simulink model "CDPR_simulation"  (R2021b)
settings: Solver=VariableStepAuto  StartTime=0.0  StopTime=40.0  RelTol=1e-3
values from neighbouring files (symbols this model uses):
  a = [-2.0 2.0 ... (first row only)    [init.m]
  A_p = [0  1   0  0   0  0 ... (first row only)    [init.m]
  b = [-0.05  0.05 ... (first row only)    [init.m]
  B_p = [0     0     0 ... (first row only)    [init.m]
  Clarke = 2/3*[1 -1/2       -1/2 ... (first row only)    [motor_init.m]
  epsilon_1 = 1e-17    [init.m]
  epsilon_2 = 1e-17    [init.m]
  f_max = 60*ones(m,1)    [init.m]
  f_min = 2*ones(m,1)    [init.m]
  f_ref = 0.5*(f_min+f_max)    [init.m]
  fourier_coeff_a = [ 0.08333    0.00000     0.00000 ... (first row only)    [motor_init.m]
  fourier_coeff_b = [-1.23020    0.60792     0.60792 ... (first row only)    [motor_init.m]
  J_m_inv = 1000*1/J_m    (= 41564.487302)    [motor_init.m]
  K_e = 0.052    [motor_init.m]
  k_spring = diag(200*ones(m,1))    [init.m]
  k_spring_inv = inv(k_spring)    [init.m]
  l_0 = inverseKinematics(a, b, x, m)    [init.m]
  L_m = 8.97e-6    (= 8.97e-06)    [motor_init.m]
  m = 4    [init.m]
  n_pole_pairs = n_poles/2    (= 7)    [motor_init.m]
  R_m = 19.00e-3    (= 0.019)    [motor_init.m]
  r_winch = 60.0e-3    (= 0.06)    [init.m]
  tau = 1e-6    (= 1e-06)    [init.m]
  theta_r_0 = (l_0-k_spring_inv*f_ref)/r_winch    [init.m]
  x_0 = [x(1); 0; x(2); 0; x(3);0]    [init.m]
  xi = 2    [init.m]
(part 2 of 2)

== matlab function CDPR_simulation/Inverse kinematics2/Inverse kinematics ==
  data: a input; l output; b input; pose input; m input
function l = inverseKinematics(a, b, pose, m)
    x     = pose(1);
    y     = pose(2);
    theta = pose(3);

    l = zeros(4,1);
    for i=1:m
        l(i) = norm(a(:,i)-[x;y]-R_z(theta)*b(:,i),2);
    end
end


function R = R_z(theta)
    R = [cos(theta) -sin(theta);
         sin(theta)  cos(theta)];
end

== matlab function CDPR_simulation/Inverse kinematics/Inverse kinematics ==
  data: a input; l output; b input; pose input; m input
function l = inverseKinematics(a, b, pose, m)
    x     = pose(1);
    y     = pose(2);
    theta = pose(3);

    l = zeros(4,1);
    for i=1:m
        l(i) = norm(a(:,i)-[x;y]-R_z(theta)*b(:,i),2);
    end
end


function R = R_z(theta)
    R = [cos(theta) -sin(theta);
         sin(theta)  cos(theta)];
end

== matlab function CDPR_simulation/Structure matrix/Structure matrix calculation ==
  data: u input; A_T output; pose input; b input; m input
function A_T = calculateStructureMatrix(u, pose, b, m)
    theta = pose(3);
    crossProd = zeros(1, 4);
    for i=1:m
        b_rot = R_z(theta)*b(:,i);
        crossProd(i) = b_rot(1)*u(2,i) - b_rot(2)*u(1,i);
    end
    A_T = [u; crossProd]
end

function R = R_z(theta)
    R = [cos(theta) -sin(theta);
         sin(theta)  cos(theta)];
end

== matlab function CDPR_simulation/Motor 1/FOC BLDC/BLDC motor/Subsystem/MATLAB Function ==
  data: a_f input; f_abc output; b_f input; theta_r input
function f_abc  = normalized_back_EMF(a_f,b_f,theta_r)
sa = 0;
sb = 0;
sc = 0;
ca = 0;
cb = 0;
cc = 0;
n = size(a_f,1);

for i = 1:n
%     ca = ca + a(i,1)*cos((i-1)*theta_r);
    cb = cb + a_f(i,2)*cos((i-1)*theta_r);
    cc = cc + a_f(i,3)*cos((i-1)*theta_r); 
end
for i = 1:2:n
    sa = sa + b_f(i,1)*sin(i*theta_r);
    sb = sb + b_f(i,2)*sin(i*theta_r);
    sc = sc + b_f(i,3)*sin(i*theta_r);
end
f_a = ca+sa;
f_b = cb+sb;
f_c = cc+sc;

f_abc = [f_a;f_b;f_c];

== matlab function CDPR_simulation/Motor 1/FOC BLDC/Inverse Park transformation ==
  data: v_q input; v_d input; v_a output; theta_r input; v_b output; v_c output
function [v_a, v_b, v_c] = inverse_park(v_q, v_d, theta_r)
Park_inv = [cos(theta_r)          -sin(theta_r);
            cos(theta_r - 2*pi/3) -sin(theta_r - 2*pi/3);
            cos(theta_r + 2*pi/3) -sin(theta_r + 2*pi/3)];

v_abc = Park_inv*[v_d;v_q];

v_a = v_abc(1);
v_b = v_abc(2);
v_c = v_abc(3);

== matlab function CDPR_simulation/Motor 1/FOC BLDC/Park transformation ==
  data: i_alphabeta input; i_qd output; theta_r input
function i_qd = park(i_alphabeta, theta_r)
Park = [-sin(theta_r) cos(theta_r);
         cos(theta_r) sin(theta_r)];
i_qd = Park*i_alphabeta;

== matlab function CDPR_simulation/Force distribution/Force distribution calculation ==
  data: A_T input; f input; f_d output; f_min input; f_max input; f_ref input; w input; m input
function f_d = forceQP(A_T, f, f_min, f_max, f_ref, w, m)
    coder.extrinsic('quadprog');
    coder.extrinsic('optimoptions');
    options = optimoptions('quadprog','Display','off');
    f_d = zeros(4,1);
%     f
%     A_T
%     f_min
%     f_max
%     f_ref
%     w
    f_d = quadprog(eye(m),-f_ref,[],[],A_T, -w,f_min,f_max, f, options);

== matlab function CDPR_simulation/Force distribution/MATLAB Function ==
  data: A_T input; f_d output; w input; f_min input; f_max input
function f_d = fcn(A_T, w, f_min, f_max)
A_T_Pinv = pinv(A_T);
f_ref = (f_min + f_max)/2;
f_d = f_ref - A_T_Pinv*(w + A_T*f_ref);
%  = u;

== matlab function CDPR_simulation/Motor 2/FOC BLDC/BLDC motor/Subsystem/MATLAB Function ==
  data: a_f input; f_abc output; b_f input; theta_r input
function f_abc  = normalized_back_EMF(a_f,b_f,theta_r)
sa = 0;
sb = 0;
sc = 0;
ca = 0;
cb = 0;
cc = 0;
n = size(a_f,1);

for i = 1:n
%     ca = ca + a(i,1)*cos((i-1)*theta_r);
    cb = cb + a_f(i,2)*cos((i-1)*theta_r);
    cc = cc + a_f(i,3)*cos((i-1)*theta_r); 
end
for i = 1:2:n
    sa = sa + b_f(i,1)*sin(i*theta_r);
    sb = sb + b_f(i,2)*sin(i*theta_r);
    sc = sc + b_f(i,3)*sin(i*theta_r);
end
f_a = ca+sa;
f_b = cb+sb;
f_c = cc+sc;

f_abc = [f_a;f_b;f_c];
